simulink model "dVOC_control_demo_fault_2023b_constDC"  (R2023b)
settings: Solver=ode23tb  StartTime=0.0  StopTime=Tend  RelTol=1e-3
values from neighbouring files (symbols this model uses):
  alpha = 1e-1*V_m^2    [dVOC_control_Psensitivity.m]    (also in dVOC_control_demo.m)
  C_4 = 0.1670*C_b    (= 1.00487241952e-06)    [dVOC_control_Psensitivity.m]    (also in dVOC_control_demo.m)
  C_8 = 0.2275*C_b    (= 1.36891302659e-06)    [dVOC_control_Psensitivity.m]    (also in dVOC_control_demo.m)
  C_dc = 0.008*(n)    (= 1.6)    [dVOC_control_Psensitivity.m]    (also in dVOC_control_demo.m)
  C_f = n*300*10^-6    (= 0.06)    [dVOC_control_Psensitivity.m]    (also in dVOC_control_demo.m)
  droop_percentage = 1    [dVOC_control_Psensitivity.m]    (also in dVOC_control_demo.m)
  eta = m_p*V_m^2    [dVOC_control_Psensitivity.m]    (also in dVOC_control_demo.m)
  i_ll = -1.15*(S_b/Vdc_n)-i_loss_dc    [dVOC_control_Psensitivity.m]    (also in dVOC_control_demo.m)
  i_ul = 1.15*(S_b/Vdc_n)+i_loss_dc    [dVOC_control_Psensitivity.m]    (also in dVOC_control_demo.m)
  k_dc = eta_1/(Vdc_n*m_p)    [dVOC_control_Psensitivity.m]    (also in dVOC_control_demo.m)
  K_p = (1/Vdc_n)    [dVOC_control_Psensitivity.m]    (also in dVOC_control_demo.m)
  K_r = 1/R_dc    [dVOC_control_Psensitivity.m]    (also in dVOC_control_demo.m)
  Kff_i = 1    [dVOC_control_Psensitivity.m]    (also in dVOC_control_demo.m)
  Kff_v = 1    [dVOC_control_Psensitivity.m]    (also in dVOC_control_demo.m)
  Ki_i = (1/n)*1.19    (= 0.00595)    [dVOC_control_Psensitivity.m]    (also in dVOC_control_demo.m)
  Ki_v = (n)*1.161022    (= 232.2044)    [dVOC_control_Psensitivity.m]    (also in dVOC_control_demo.m)
  Kp_i = 0.738891    [dVOC_control_Psensitivity.m]    (also in dVOC_control_demo.m)
  Kp_v = 0.52    [dVOC_control_Psensitivity.m]    (also in dVOC_control_demo.m)
  L1_pu = 1*0.0186/m    (= 0.000186)    [dVOC_control_Psensitivity.m]    (also in dVOC_control_demo.m)
  L_45 = L_lines(2)    [dVOC_control_Psensitivity.m]    (also in dVOC_control_demo.m)
  L_89 = L_lines(8)    [dVOC_control_Psensitivity.m]    (also in dVOC_control_demo.m)
  L_94 = L_lines(9)    [dVOC_control_Psensitivity.m]    (also in dVOC_control_demo.m)
  L_f = (1/n)*200*10^-6    (= 1e-06)    [dVOC_control_Psensitivity.m]    (also in dVOC_control_demo.m)
  n = 200    [dVOC_control_Psensitivity.m]    (also in dVOC_control_demo.m)
  pl = S_b*ps    (= 75000000)    [dVOC_control_Psensitivity.m]    (also in dVOC_control_demo.m)
  ps = base/3    (= 0.75)    [dVOC_control_Psensitivity.m]    (also in dVOC_control_demo.m)
  qs = [0;0]    [dVOC_control_Psensitivity.m]    (also in dVOC_control_demo.m)
  R1_pu = 1*0.00734/m    (= 7.34e-05)    [dVOC_control_Psensitivity.m]    (also in dVOC_control_demo.m)
  R_45 = R_lines(2)    [dVOC_control_Psensitivity.m]    (also in dVOC_control_demo.m)
  R_89 = R_lines(8)    [dVOC_control_Psensitivity.m]    (also in dVOC_control_demo.m)
  R_94 = R_lines(9)    [dVOC_control_Psensitivity.m]    (also in dVOC_control_demo.m)
  R_dc = (Vdc_n/(0.05*(S_b)/Vdc_n))    [dVOC_control_Psensitivity.m]    (also in dVOC_control_demo.m)
  R_f = 0.001/n    (= 5e-06)    [dVOC_control_Psensitivity.m]    (also in dVOC_control_demo.m)
  S_b = 100*(10^6)    (= 100000000)    [dVOC_control_Psensitivity.m]    (also in dVOC_control_demo.m)
  S_bt = S_b    (= 100000000)    [dVOC_control_Psensitivity.m]    (also in dVOC_control_demo.m)
  t_disturbance = linspace(0.01,0.2,10)    [dVOC_control_Psensitivity.m]    (also in dVOC_control_demo.m; data_post_process_ExtendSmooth.m = 5+linspace(0.01,0.2,n_period); data_post_process_ExtendSmooth_Psensitivity.m = 5+linspace(0.0,0.0,n_period))
  T_en = T_load(1)-0.5    [dVOC_control_Psensitivity.m]    (also in dVOC_control_demo.m)
  T_load = [5 5]    [dVOC_control_Psensitivity.m]    (also in dVOC_control_demo.m = [5 5.2])
  T_load1 = [T_load(1)-dt_load(1), T_load(1)]    [dVOC_control_Psensitivity.m]    (also in dVOC_control_demo.m = [T_load(1), T_load(1) + dt_load(1)])
  T_load2 = [T_load(1)-dt_load(2), T_load(1)]    [dVOC_control_Psensitivity.m]    (also in dVOC_control_demo.m = [T_load(1), T_load(1) + dt_load(2)])
  T_loss = Tend    (= 8)    [dVOC_control_Psensitivity.m]    (also in dVOC_control_demo.m)
  T_s = 3.125e-4/4    (= 7.8125e-05)    [dVOC_control_Psensitivity.m]    (also in dVOC_control_demo.m)
  tau_dc = 0.05    [dVOC_control_Psensitivity.m]    (also in dVOC_control_demo.m)
  tau_g = 5    [dVOC_control_Psensitivity.m]    (also in dVOC_control_demo.m)
  V1_rms = 1000    [dVOC_control_Psensitivity.m]    (also in dVOC_control_demo.m)
  V2_rms = 13800    [dVOC_control_Psensitivity.m]    (also in dVOC_control_demo.m)
  V_m = sqrt(2/3)*V1_rms    [dVOC_control_Psensitivity.m]    (also in dVOC_control_demo.m)
  Vdc_n = 3*V_m    [dVOC_control_Psensitivity.m]    (also in dVOC_control_demo.m)
  w_b = 2*pi*f_b    (= 314.159265359)    [dVOC_control_Psensitivity.m]    (also in dVOC_control_demo.m)
  w_f = 2*pi*5    (= 31.4159265359)    [dVOC_control_Psensitivity.m]    (also in dVOC_control_demo.m)
undefined symbols (not defined in the file or in its folder): D1, Delta, i_dc, i_t
libraries: eePMU x12, simulink_extras x9, spsabctoAlphaBetaZeroLib x9, spsSeriesRLCBranchLib x8, spsVoltageMeasurementLib x7, spsThreePhaseVIMeasurementLib x6, spsCurrentMeasurementLib x6, spsabctodq0Lib x6, spsGroundLib x5, spsThreePhaseParallelRLCLoadLib x3, spsThreePhaseBreakerLib x3, cstblocks x3
(part 1 of 2)
settings Model: ExtModeTrigDuration=100  Creator=TayyebiA  LastModifiedBy=lab-admin
settings SolverCC: AlgebraicLoopSolver=TrustRegion
settings DataIOCC: SaveFormat=StructureWithTime  SaveOutput=off  ReturnWorkspaceOutputs=off  StateSaveName=tmp_raccel_xout  SignalLoggingName=tmp_raccel_logsout
settings OptimizationCC: EfficientMapNaN2IntZero=off
settings DebuggingCC: AlgebraicLoopMsg=none  ArithmeticOperatorsInVariantConditions=warning
settings HardwareCC: TargetBitPerLong=64  TargetBitPerPointer=64  TargetBitPerSizeT=64  TargetBitPerPtrDiffT=64  TargetLongLongMode=on  TargetIntDivRoundTo=Zero  TargetEndianess=LittleEndian  TargetWordSize=64  TargetHWDeviceType=MATLAB Host  ProdEqTarget=off
settings ModelReferenceCC: EnableRefExpFcnMdlSchedulingChecks=on
settings SFSimCC: SimUseLocalCustomCode=off  CustomCodeUndefinedFunction=UseInterfaceOnly
settings RTWCC: RTWUseLocalCustomCode=off
settings CodeAppCC: MaxIdLength=128
settings GRTTargetCC: TargetLangStandard=C89/C90 (ANSI)  CombineOutputUpdateFcns=off  GRTInterface=on

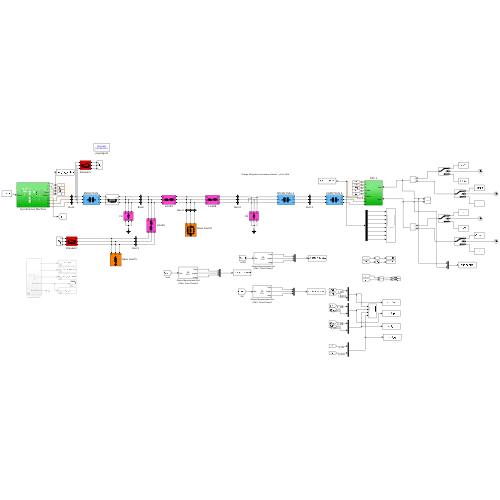
[thumbnail: Simulink's stored preview of the top-level diagram]
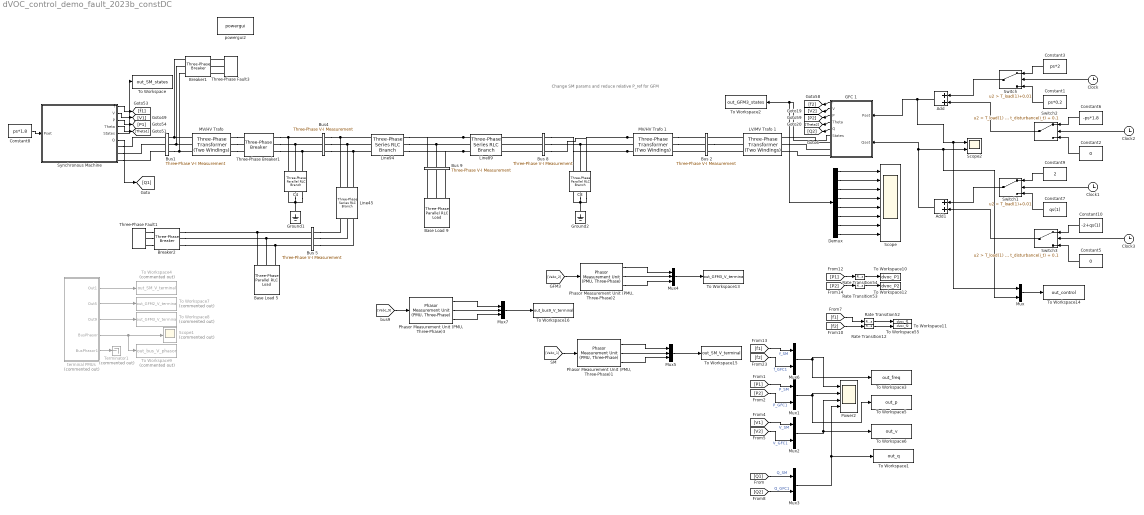
== system dVOC_control_demo_fault_2023b_constDC ==
  note: Change SM params and reduce relative P_ref for GFM
  Add : Sum
  Add1 : Sum
  Base Load 5 : spsThreePhaseParallelRLCLoadLib/Three-Phase Parallel RLC Load  LConnTagsString=A|B|C  Configuration=Y (grounded)  NominalVoltage=230e3  Vabc=[1e3 1e3 1e3]  Vabcp=[1e3 1e3 1e3]  NominalFrequency=50  UnbalancedPower=off  ActivePower=pl  InductivePower=0  CapacitivePower=0  Pabc=[10e3 9e3 11e3]  QLabc=[100 90 110]  QCabc=[100 90 110]  Pabcp=[10e3 9e3 11e3]  QLabcp=[100 90 110]  QCabcp=[100 90 110]  Measurements=None  LoadType=constant Z
  "Base Load 9 " : spsThreePhaseParallelRLCLoadLib/Three-Phase Parallel RLC Load  LConnTagsString=A|B|C  Configuration=Y (grounded)  NominalVoltage=230e3  Vabc=[1e3 1e3 1e3]  Vabcp=[1e3 1e3 1e3]  NominalFrequency=50  UnbalancedPower=off  ActivePower=pl  InductivePower=1*pl  CapacitivePower=1*pl  Pabc=[10e3 9e3 11e3]  QLabc=[100 90 110]  QCabc=[100 90 110]  Pabcp=[10e3 9e3 11e3]  QLabcp=[100 90 110]  QCabcp=[100 90 110]  Measurements=None  LoadType=constant PQ
  Breaker1 : spsThreePhaseBreakerLib/Three-Phase Breaker  InitialState=open  SwitchA=on  SwitchB=on  SwitchC=on  SwitchTimes=[T_load2]  External=off  BreakerResistance=0.01  SnubberResistance=1e6  SnubberCapacitance=inf  Measurements=None
  Breaker2 : spsThreePhaseBreakerLib/Three-Phase Breaker  InitialState=open  SwitchA=on  SwitchB=on  SwitchC=on  SwitchTimes=[T_load1]  External=off  BreakerResistance=0.01  SnubberResistance=1e6  SnubberCapacitance=inf  Measurements=None
  Bus 2 : spsThreePhaseVIMeasurementLib/Three-Phase V-I Measurement  VoltageMeasurement=phase-to-ground  SetLabelV=on  LabelV=Vabc_2  Vpu=on  VpuLL=off  CurrentMeasurement=no  SetLabelI=on  LabelI=Iabc_8  Ipu=on  Pbase=S_b  Vbase=V2_rms  OutputType=Complex  PhasorSimulation=off  PSBequivalent=0
  Bus 5 : spsThreePhaseVIMeasurementLib/Three-Phase V-I Measurement  VoltageMeasurement=phase-to-ground  SetLabelV=on  LabelV=Vabc_5  Vpu=on  VpuLL=off  CurrentMeasurement=no  SetLabelI=on  LabelI=Iabc_5  Ipu=on  Pbase=S_b  Vbase=V_b  OutputType=Complex  PhasorSimulation=off  PSBequivalent=0
  Bus 8 : spsThreePhaseVIMeasurementLib/Three-Phase V-I Measurement  VoltageMeasurement=phase-to-ground  SetLabelV=on  LabelV=Vabc_8  Vpu=on  VpuLL=off  CurrentMeasurement=no  SetLabelI=on  LabelI=Iabc_8  Ipu=on  Pbase=S_b  Vbase=V_b  OutputType=Complex  PhasorSimulation=off  PSBequivalent=0
  Bus 9 : spsThreePhaseVIMeasurementLib/Three-Phase V-I Measurement  VoltageMeasurement=phase-to-ground  SetLabelV=on  LabelV=Vabc_9  Vpu=on  VpuLL=off  CurrentMeasurement=no  SetLabelI=on  LabelI=Iabc_9  Ipu=on  Pbase=S_b  Vbase=V_b  OutputType=Complex  PhasorSimulation=off  PSBequivalent=0
  Bus1 : spsThreePhaseVIMeasurementLib/Three-Phase V-I Measurement  VoltageMeasurement=phase-to-ground  SetLabelV=on  LabelV=Vabc_1  Vpu=on  VpuLL=off  CurrentMeasurement=no  SetLabelI=on  LabelI=Iabc_1  Ipu=on  Pbase=S_b  Vbase=V2_rms  OutputType=Complex  PhasorSimulation=off  PSBequivalent=0
  Bus4 : spsThreePhaseVIMeasurementLib/Three-Phase V-I Measurement  VoltageMeasurement=phase-to-ground  SetLabelV=on  LabelV=Vabc_4  Vpu=on  VpuLL=off  CurrentMeasurement=no  SetLabelI=on  LabelI=Iabc_4  Ipu=on  Pbase=S_b  Vbase=V_b  OutputType=Complex  PhasorSimulation=off  PSBequivalent=0
  C4 : spsThreePhaseParallelRLCBranchLib/Three-Phase Parallel RLC Branch  LConnTagsString=A|B|C  RConnTagsString=A|B|C  BranchType=C  Resistance=1  Inductance=1e-3  Capacitance=C_4  Measurements=None
  C8 : spsThreePhaseParallelRLCBranchLib/Three-Phase Parallel RLC Branch  LConnTagsString=A|B|C  RConnTagsString=A|B|C  BranchType=C  Resistance=1  Inductance=1e-3  Capacitance=C_8  Measurements=None
  Clock{,1..3} (4 alike) : Clock
      settings: Decimation=5
  Constant1 : Constant  Value=ps*0.2
  Constant10 : Constant  Value=-2+qs(1)
  Constant2 : Constant  Value=0
  Constant3 : Constant  Value=ps*2
  Constant5 : Constant  Value=0
  Constant6 : Constant  Value=-ps*1.8
  Constant7 : Constant  Value=qs(1)
  Constant8 : Constant  Value=ps*1.8
  Constant9 : Constant  Value=2
  Demux : Demux  Outputs=8
  GFC 1 : Subsystem
  Ground1 : spsGroundLib/Ground  LConnTagsString=a
  Ground2 : spsGroundLib/Ground  LConnTagsString=a
  LV/MV Trafo 1 : spsThreePhaseTransformerTwoWindingsLib/Three-Phase Transformer (Two Windings)  Winding1Connection=Yg  Winding2Connection=Yg  CoreType=Three single-phase transformers  SetSaturation=off  Hysteresis=off  DataFile='hysteresis'  SetInitialFlux=off  Measurements=None  UNITS=pu  NominalPower=[S_bt 50 ]  Winding1="[ V1_rms R1_pu  L1_pu]"  Winding2=[ V2_rms R1_pu L1_pu]  Rm=Rm_pu  Lm=Lm_pu  L0=0.5  Saturation="[ 0,0  ;  0.005,1.2  ;  1.0,1.4 ]"  InitialFluxes=[ 0.8 , -0.8 , 0.7 ]  BreakLoop=off  DiscreteSolver=Trapezoidal iterative  DataType=off  TransfoNumber=0
  Line45 : spsThreePhaseSeriesRLCBranchLib/Three-Phase Series RLC Branch  LConnTagsString=A|B|C  RConnTagsString=A|B|C  BranchType=RL  Resistance=R_45  Inductance=L_45  Capacitance=0  Measurements=None
  Line89 : spsThreePhaseSeriesRLCBranchLib/Three-Phase Series RLC Branch  LConnTagsString=A|B|C  RConnTagsString=A|B|C  BranchType=RL  Resistance=R_89  Inductance=L_89  Capacitance=0  Measurements=None
  Line94 : spsThreePhaseSeriesRLCBranchLib/Three-Phase Series RLC Branch  LConnTagsString=A|B|C  RConnTagsString=A|B|C  BranchType=RL  Resistance=R_94  Inductance=L_94  Capacitance=0  Measurements=None
  "MV/HV Trafo " : spsThreePhaseTransformerTwoWindingsLib/Three-Phase Transformer (Two Windings)  Winding1Connection=Delta (D1)  Winding2Connection=Yg  CoreType=Three single-phase transformers  SetSaturation=off  Hysteresis=off  DataFile='hysteresis'  SetInitialFlux=off  Measurements=None  UNITS=pu  NominalPower=[ 210e6 50 ]  Winding1="[V2_rms 0.0027  0.08]"  Winding2=[230e3 0.0027 0.08]  Rm=500  Lm=500  L0=0.5  Saturation="[ 0,0  ;  0.005,1.2  ;  1.0,1.4 ]"  InitialFluxes=[ 0.8 , -0.8 , 0.7 ]  BreakLoop=off  DiscreteSolver=Trapezoidal iterative  DataType=off  TransfoNumber=0
  "MV/HV Trafo 1 " : spsThreePhaseTransformerTwoWindingsLib/Three-Phase Transformer (Two Windings)  Winding1Connection=Yg  Winding2Connection=Yg  CoreType=Three single-phase transformers  SetSaturation=off  Hysteresis=off  DataFile='hysteresis'  SetInitialFlux=off  Measurements=None  UNITS=pu  NominalPower=[ 210e6 50 ]  Winding1=[V2_rms 0.0027 0.08]  Winding2=[ 230e3 0.0027 0.08]  Rm=500  Lm=500  L0=0.5  Saturation="[ 0,0  ;  0.005,1.2  ;  1.0,1.4 ]"  InitialFluxes=[ 0.8 , -0.8 , 0.7 ]  BreakLoop=off  DiscreteSolver=Trapezoidal iterative  DataType=off  TransfoNumber=0
  Mux{,1..3,6} (5 alike) : Mux  Inputs=2
  Mux4 : Mux  Inputs=3
  Mux5 : Mux  Inputs=3
  Mux7 : Mux  Inputs=3
  "Phasor Measurement Unit (PMU, Three-Phase)1" : eePMU/Phasor Measurement Unit (PMU, Three-Phase)  frequency=50  Nsr=64  k=1
      settings: LibrarySourceBlock=|
      | ee_sl_lib/Measurements/Phasor Measurement Unit
      | (PMU, Three-Phase)
  "Phasor Measurement Unit (PMU, Three-Phase)2" : eePMU/Phasor Measurement Unit (PMU, Three-Phase)  frequency=50  Nsr=64  k=1
      settings: LibrarySourceBlock=|
      | ee_sl_lib/Measurements/Phasor Measurement Unit
      | (PMU, Three-Phase)
  "Phasor Measurement Unit (PMU, Three-Phase)3" : eePMU/Phasor Measurement Unit (PMU, Three-Phase)  frequency=50  Nsr=64  k=1
      settings: LibrarySourceBlock=|
      | ee_sl_lib/Measurements/Phasor Measurement Unit
      | (PMU, Three-Phase)
  Power2 : Scope  NumInputPorts=4
  Rate Transition{12,52..54} (4 alike) : RateTransition  OutPortSampleTime=T_ms
  Scope : Scope  NumInputPorts=8
  Scope1 : Scope  Commented=on
  Scope2 : Scope  NumInputPorts=2
  Switch : Switch  Criteria=u2 > Threshold  Threshold=T_load(1)+0.01  SaturateOnIntegerOverflow=off  InputSameDT=off
  Switch1 : Switch  Criteria=u2 > Threshold  Threshold=T_load(1)+0.01  SaturateOnIntegerOverflow=off  InputSameDT=off
  Switch2 : Switch  Criteria=u2 > Threshold  Threshold=T_load(1) + t_disturbance(i_t) + 0.1  SaturateOnIntegerOverflow=off  InputSameDT=off
  Switch3 : Switch  Criteria=u2 > Threshold  Threshold=T_load(1) + t_disturbance(i_t) + 0.1  SaturateOnIntegerOverflow=off  InputSameDT=off
  Synchronous Machine : Subsystem
  Terminator1 : Terminator  Commented=on
  Three-Phase Breaker1 : spsThreePhaseBreakerLib/Three-Phase Breaker  InitialState=closed  SwitchA=on  SwitchB=on  SwitchC=on  SwitchTimes=[T_loss]  External=off  BreakerResistance=1  SnubberResistance=1e6  SnubberCapacitance=inf  Measurements=None
  Three-Phase Fault1 : spsThreePhaseFaultLib/Three-Phase Fault  InitialStates=0  FaultA=on  FaultB=on  FaultC=on  GroundFault=on  SwitchTimes=[T_load1]  External=off  SwitchStatus=NaN  FaultResistance=0.001  GroundResistance=0.01  SnubberResistance=1e6  SnubberCapacitance=inf  Measurements=None
  Three-Phase Fault3 : spsThreePhaseFaultLib/Three-Phase Fault  InitialStates=0  FaultA=on  FaultB=on  FaultC=on  GroundFault=on  SwitchTimes=[T_load2]  External=off  SwitchStatus=NaN  FaultResistance=0.001  GroundResistance=0.01  SnubberResistance=1e6  SnubberCapacitance=inf  Measurements=None
  To Workspace : ToWorkspace  VariableName=out_SM_states  SaveFormat=Timeseries  SampleTime=-1
  To Workspace1 : ToWorkspace  VariableName=out_q  SaveFormat=Timeseries  SampleTime=-1
  To Workspace10 : ToWorkspace  VariableName=dvoc_P1  SampleTime=-1
  To Workspace11 : ToWorkspace  VariableName=dvoc_f2  SampleTime=-1
  To Workspace12 : ToWorkspace  VariableName=dvoc_P2  SampleTime=-1
  To Workspace13 : ToWorkspace  VariableName=out_GFM3_V_terminal  SaveFormat=Timeseries  SampleTime=-1
  To Workspace14 : ToWorkspace  VariableName=out_control  SaveFormat=Timeseries  SampleTime=-1
  To Workspace15 : ToWorkspace  VariableName=out_SM_V_terminal  SaveFormat=Timeseries  SampleTime=-1
  To Workspace16 : ToWorkspace  VariableName=out_bus9_V_terminal  SaveFormat=Timeseries  SampleTime=-1
  To Workspace2 : ToWorkspace  VariableName=out_GFM3_states  SaveFormat=Timeseries  SampleTime=-1
  To Workspace3 : ToWorkspace  VariableName=out_freq  SaveFormat=Timeseries  SampleTime=-1
  To Workspace4 : ToWorkspace  Commented=on  VariableName=out_SM_V_terminal  SaveFormat=Timeseries  SampleTime=-1
  To Workspace5 : ToWorkspace  VariableName=out_p  SaveFormat=Timeseries  SampleTime=-1
  To Workspace55 : ToWorkspace  VariableName=dvoc_f1  SampleTime=-1
  To Workspace6 : ToWorkspace  VariableName=out_v  SaveFormat=Timeseries  SampleTime=-1
  To Workspace7 : ToWorkspace  Commented=on  VariableName=out_GFM2_V_terminal  SaveFormat=Timeseries  SampleTime=-1
  To Workspace8 : ToWorkspace  Commented=on  VariableName=out_GFM3_V_terminal  SaveFormat=Timeseries  SampleTime=-1
  To Workspace9 : ToWorkspace  Commented=on  VariableName=out_bus_V_phasor  SaveFormat=Timeseries  SampleTime=-1
  powergui2 : sps_lib/powergui  Priority=1  SimulationMode=Discrete  SampleTime=T_s  frequency=50  Iterations=50  frequencyindice=0  Pbase=100e6  ErrMax=0.0001  UnitsV=kV  UnitsW=MW  buscounter=0  FunctionMessages=off  echomessages=off  EnableUseOfTLC=off  CurrentSourceSwitches=off  DisableSnubberDevices=off  DisableRonSwitches=off  DisableVfSwitches=off  DisplayEquations=off  AutomaticDiscreteSolvers=off  SolverType=Tustin/Backward Euler (TBE)  Interpol=off  ExternalGateDelay=off  methode=off  Ts=100  x0status=blocks  SPID=off  SwTol=0  HookPort=off  NonlinearTolerance=1e-4  nMaxIteration=100  ContinueOnMaxIteration=off  RestoreLinks=warning  ResistiveCurrentMeasurement=off  Frange=[0:2:500]  Ylog=off  Xlog=on  ShowGrid=off  save=off  variable=ZData  structure=0  ZoomFFT=off  StartTime=0.0  cycles=1  DisplayStyle=1  fundamental=60  FreqAxis=off  MaxFrequency=1000  frequencyindicesteady=1  RmsSteady=1  display=off
  terminal PMUs : Subsystem  Commented=on
  wires:
  Constant8/1 -> Synchronous Machine/1(Pset)
  Synchronous Machine/1(f) -> [f1]
  Synchronous Machine/2(V) -> [V1]
  Synchronous Machine/3(P) -> [P1]
  Synchronous Machine/4(Theta) -> [Theta1]
  [f1] -> Mux6/1  "f_SM"
  [f2] -> Mux6/2  "f_GFC1"
  [P1] -> Mux1/1  "P_SM"
  [P2] -> Mux1/2  "P_GFC1"
  [V2] -> Mux2/2  "V_GFC1"
  [V1] -> Mux2/1  "V_SM"
  Mux6/1 -> Power2/1, To Workspace3/1
  Mux1/1 -> Power2/2, To Workspace5/1
  Mux2/1 -> To Workspace6/1, Power2/3
  GFC 1/1(f) -> [f2]
  GFC 1/2(V) -> [V2]
  GFC 1/3(P) -> [P2]
  GFC 1/4(Theta) -> [Theta2]
  GFC 1/5(Q) -> [Q2]
  Mux3/1 -> To Workspace1/1, Power2/4
  [Q2] -> Mux3/2  "Q_GFC1"
  Rate Transition12/1 -> To Workspace11/1
  Rate Transition53/1 -> To Workspace12/1
  Rate Transition54/1 -> To Workspace10/1
  Rate Transition52/1 -> To Workspace55/1
  [f1] -> Rate Transition52/1
  [f2] -> Rate Transition12/1
  [P2] -> Rate Transition53/1
  [P1] -> Rate Transition54/1
  terminal PMUs/3(Out9) -> To Workspace8/1
  terminal PMUs/1(Out1) -> To Workspace4/1
  terminal PMUs/2(Out5) -> To Workspace7/1
  Synchronous Machine/5(States) -> To Workspace/1
  GFC 1/6(States) -> To Workspace2/1, Demux/1
  Demux/1 -> Scope/1
  Demux/2 -> Scope/2
  Demux/3 -> Scope/3
  Demux/4 -> Scope/4
  Demux/5 -> Scope/5
  Demux/6 -> Scope/6
  Demux/7 -> Scope/7
  Demux/8 -> Scope/8
  terminal PMUs/4(BusPhasor) -> To Workspace9/1, Scope1/1
  terminal PMUs/5(BusPhasor1) -> Terminator1/1
  Clock/1 -> Switch/2
  Constant3/1 -> Switch/1
  Constant1/1 -> Switch/3
  Synchronous Machine/6(Q) -> [Q1]
  [Q1] -> Mux3/1  "Q_SM"
  Clock2/1 -> Switch2/2
  Constant2/1 -> Switch2/3
  Constant6/1 -> Switch2/1
  Add/1 -> Mux/1, Scope2/1, GFC 1/1(Pset)
  Switch/1 -> Add/1
  Switch2/1 -> Add/2
  Constant5/1 -> Switch3/3
  Add1/1 -> Mux/2, Scope2/2, GFC 1/2(Qset)
  Switch1/1 -> Add1/1
  Clock3/1 -> Switch3/2
  Switch3/1 -> Add1/2
  Constant10/1 -> Switch3/1
  Constant7/1 -> Switch1/3
  Clock1/1 -> Switch1/2
  Constant9/1 -> Switch1/1
  "Phasor Measurement Unit (PMU, Three-Phase)2"/2 -> Mux4/2
  [Vabc_2] -> "Phasor Measurement Unit (PMU, Three-Phase)2"/1
  "Phasor Measurement Unit (PMU, Three-Phase)2"/1 -> Mux4/1
  "Phasor Measurement Unit (PMU, Three-Phase)2"/3 -> Mux4/3
  Mux4/1 -> To Workspace13/1
  Mux/1 -> To Workspace14/1
  "Phasor Measurement Unit (PMU, Three-Phase)1"/2 -> Mux5/2
  "Phasor Measurement Unit (PMU, Three-Phase)1"/1 -> Mux5/1
  [Vabc_1] -> "Phasor Measurement Unit (PMU, Three-Phase)1"/1
  "Phasor Measurement Unit (PMU, Three-Phase)1"/3 -> Mux5/3
  Mux5/1 -> To Workspace15/1
  "Phasor Measurement Unit (PMU, Three-Phase)3"/2 -> Mux7/2
  [Vabc_9] -> "Phasor Measurement Unit (PMU, Three-Phase)3"/1
  Mux7/1 -> To Workspace16/1
  "Phasor Measurement Unit (PMU, Three-Phase)3"/3 -> Mux7/3
  "Phasor Measurement Unit (PMU, Three-Phase)3"/1 -> Mux7/1
  connections:
  Bus 8/RConn2 -- Line89/RConn2
  "MV/HV Trafo 1 "/RConn3 -- C8/LConn3 -- Bus 8/LConn3
  Line94/RConn2 -- Bus 9/RConn2 -- Line89/LConn2
  Bus 5/LConn3 -- Line45/RConn3
  Line89/LConn1 -- Bus 9/RConn1 -- Line94/RConn1
  C4/RConn2 -- C4/RConn1 -- C4/RConn3 -- Ground1/LConn1
  "MV/HV Trafo 1 "/RConn1 -- C8/LConn1 -- Bus 8/LConn1
  Bus 8/LConn2 -- C8/LConn2 -- "MV/HV Trafo 1 "/RConn2
  C8/RConn3 -- Ground2/LConn1 -- C8/RConn2 -- C8/RConn1
  C4/LConn1 -- Bus4/RConn1 -- Three-Phase Breaker1/RConn1
  Bus4/LConn1 -- Line45/LConn1 -- Line94/LConn1
  Bus4/LConn2 -- Line45/LConn2 -- Line94/LConn2
  Bus 8/RConn3 -- Line89/RConn3
  Bus 8/RConn1 -- Line89/RConn1
  Bus4/RConn3 -- Three-Phase Breaker1/RConn3 -- C4/LConn3
  Bus 5/LConn1 -- Line45/RConn1
  Line89/LConn3 -- Bus 9/RConn3 -- Line94/RConn3
  Bus4/LConn3 -- Line45/LConn3 -- Line94/LConn3
  Bus4/RConn2 -- Three-Phase Breaker1/RConn2 -- C4/LConn2
  Bus 5/LConn2 -- Line45/RConn2
  Base Load 5/LConn3 -- Bus 5/RConn3 -- Breaker2/LConn3
  Base Load 5/LConn1 -- Bus 5/RConn1 -- Breaker2/LConn1
  Base Load 5/LConn2 -- Breaker2/LConn2 -- Bus 5/RConn2
  Bus1/LConn1 -- Breaker1/LConn1 -- "MV/HV Trafo "/LConn1
  Bus1/LConn2 -- Breaker1/LConn2 -- "MV/HV Trafo "/LConn2
  Bus1/LConn3 -- Breaker1/LConn3 -- "MV/HV Trafo "/LConn3
  Synchronous Machine/RConn1 -- Bus1/RConn1
  Synchronous Machine/RConn2 -- Bus1/RConn2
  Synchronous Machine/RConn3 -- Bus1/RConn3
  LV/MV Trafo 1/RConn3 -- Bus 2/LConn3
  "MV/HV Trafo 1 "/LConn2 -- Bus 2/RConn2
  LV/MV Trafo 1/RConn1 -- Bus 2/LConn1
  "MV/HV Trafo 1 "/LConn3 -- Bus 2/RConn3
  "MV/HV Trafo "/RConn1 -- Three-Phase Breaker1/LConn1
  "MV/HV Trafo "/RConn2 -- Three-Phase Breaker1/LConn2
  "MV/HV Trafo "/RConn3 -- Three-Phase Breaker1/LConn3
  GFC 1/RConn3 -- LV/MV Trafo 1/LConn1
  GFC 1/RConn2 -- LV/MV Trafo 1/LConn2
  GFC 1/RConn1 -- LV/MV Trafo 1/LConn3
  Three-Phase Fault1/LConn3 -- Breaker2/RConn3
  Three-Phase Fault1/LConn1 -- Breaker2/RConn1
  Three-Phase Fault1/LConn2 -- Breaker2/RConn2
  Three-Phase Fault3/LConn3 -- Breaker1/RConn3
  Three-Phase Fault3/LConn1 -- Breaker1/RConn1
  Three-Phase Fault3/LConn2 -- Breaker1/RConn2
  Bus 2/RConn1 -- "MV/HV Trafo 1 "/LConn1
  Bus 2/LConn2 -- LV/MV Trafo 1/RConn2
  "Base Load 9 "/LConn3 -- Bus 9/LConn3
  "Base Load 9 "/LConn2 -- Bus 9/LConn2
  "Base Load 9 "/LConn1 -- Bus 9/LConn1

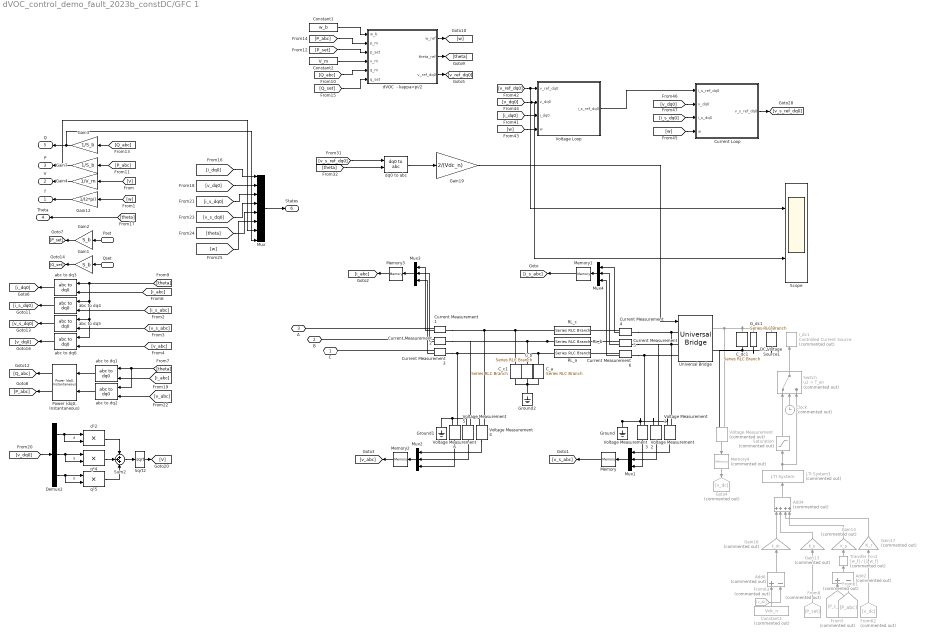
== system dVOC_control_demo_fault_2023b_constDC/GFC 1 ==
  Pset : Inport
  Qset : Inport  Port=2
  Add2 : Sum  Commented=on  Inputs=+-
  Add4 : Sum  Commented=on  Inputs=++++
  Add6 : Sum  Commented=on  Inputs=+-
  C_a : spsSeriesRLCBranchLib/Series RLC Branch  LConnTagsString=__new0  RConnTagsString=__new0  BranchType=C  Resistance=1  Inductance=1e-3  SetiL0=off  InitialCurrent=0  Capacitance=C_f  Setx0=off  InitialVoltage=165  Measurements=None
  C_b : spsSeriesRLCBranchLib/Series RLC Branch  LConnTagsString=__new0  RConnTagsString=__new0  BranchType=C  Resistance=1  Inductance=1e-3  SetiL0=off  InitialCurrent=0  Capacitance=C_f  Setx0=off  InitialVoltage=165  Measurements=None
  C_c1 : spsSeriesRLCBranchLib/Series RLC Branch  LConnTagsString=__new0  RConnTagsString=__new0  BranchType=C  Resistance=1  Inductance=1e-3  SetiL0=off  InitialCurrent=0  Capacitance=C_f  Setx0=off  InitialVoltage=165  Measurements=None
  C_dc1 : spsSeriesRLCBranchLib/Series RLC Branch  LConnTagsString=__new0  RConnTagsString=__new0  BranchType=RC  Resistance=1e-5  Inductance=1e-3  SetiL0=off  InitialCurrent=0  Capacitance=C_dc  Setx0=off  InitialVoltage=Vdc_n  Measurements=None
  Clock : Clock  Commented=on
  Constant1 : Constant  Value=w_b
  Constant2 : Constant  Value=V_m
  Constant3 : Constant  Commented=on  Value=Vdc_n
  Current Loop : Subsystem
  Current Measurement{1..6} (6 alike) : spsCurrentMeasurementLib/Current Measurement  PhasorSimulation=off  OutputType=Complex  PSBequivalent=0
  DC Voltage Source1 : spsDCVoltageSourceLib/DC Voltage Source  Amplitude=Vdc_n  Measurements=None
  Demux2 : Demux  Outputs=3
  From5 : From  Commented=on  GotoTag=P_s_abc
  From61 : From  Commented=on  GotoTag=P_abc
  From62 : From  Commented=on  GotoTag=v_dc
  From63 : From  Commented=on  GotoTag=v_dc
  From8 : From  Commented=on  GotoTag=P_set
  G_dc1 : spsSeriesRLCBranchLib/Series RLC Branch  LConnTagsString=__new0  RConnTagsString=__new0  BranchType=R  Resistance=R_dc  Inductance=1e-3  SetiL0=off  InitialCurrent=0  Capacitance=1e-6  Setx0=off  InitialVoltage=0  Measurements=None
  Gain1 : Gain  Gain=S_b
  Gain12 : Gain  Gain=1/(2*pi)
  Gain13 : Gain  Commented=on  Gain=K_p
  Gain14 : Gain  Commented=on  Gain=K_p
  Gain16 : Gain  Commented=on  Gain=k_dc
  Gain17 : Gain  Commented=on  Gain=K_r
  Gain19 : Gain  Gain=2/(Vdc_n)
  Gain2 : Gain  Gain=S_b
  Gain3 : Gain  Gain=1/S_b
  Gain4 : Gain  Gain=1/V_m
  Gain7 : Gain  Gain=1/S_b
  Goto4 : Goto  Commented=on  GotoTag=v_dc
  Ground : spsGroundLib/Ground  LConnTagsString=a
  Ground1 : spsGroundLib/Ground  LConnTagsString=a
  Ground2 : spsGroundLib/Ground  LConnTagsString=a
  LTI System3 : cstblocks/LTI System  Commented=on  sys=tf(1,[tau_dc 1])  IC=[]  PadeOrder=0
  Memory{,1..3} (4 alike) : Memory
  Memory4 : Memory  Commented=on
  Mux : Mux  Inputs=8
  Mux{1..4} (4 alike) : Mux  Inputs=3
  "Power (dq0, Instantaneous)" : spsPowerdq0InstantaneousLib/Power (dq0, Instantaneous)
      settings: LibrarySourceBlock=|
      | sps_lib/Sensors and Measurements/Power
      | (dq0, Instantaneous)
  RL_a : spsSeriesRLCBranchLib/Series RLC Branch  LConnTagsString=__new0  RConnTagsString=__new0  BranchType=RL  Resistance=R_f  Inductance=L_f  SetiL0=off  InitialCurrent=0  Capacitance=1e-6  Setx0=off  InitialVoltage=0  Measurements=Branch voltage and current
  RL_b : spsSeriesRLCBranchLib/Series RLC Branch  LConnTagsString=__new0  RConnTagsString=__new0  BranchType=RL  Resistance=R_f  Inductance=L_f  SetiL0=off  InitialCurrent=0  Capacitance=1e-6  Setx0=off  InitialVoltage=0  Measurements=None
  RL_c : spsSeriesRLCBranchLib/Series RLC Branch  LConnTagsString=__new0  RConnTagsString=__new0  BranchType=RL  Resistance=R_f  Inductance=L_f  SetiL0=off  InitialCurrent=0  Capacitance=1e-6  Setx0=off  InitialVoltage=0  Measurements=None
  Saturation : Saturate  Commented=on  UpperLimit=i_ul  LowerLimit=i_ll
  Scope : Scope  NumInputPorts=2
  Sqrt2 : Sqrt
  Sum2 : Sum  Inputs=+++  InputSameDT=on  SaturateOnIntegerOverflow=on  OutDataTypeStr=Inherit: Same as first input
  Switch : Switch  Commented=on  Criteria=u2 > Threshold  Threshold=T_en  SaturateOnIntegerOverflow=off  InputSameDT=off
  Transfer Fcn2 : TransferFcn  Commented=on  Numerator=[w_f]  Denominator=[1 w_f]
  Universal Bridge : spsUniversalBridgeLib/Universal Bridge  Arms=3  SnubberResistance=1e5  SnubberCapacitance=inf  Device=Average-model based VSC  Ron=1e-3  Lon=0  ForwardVoltages="[  0  0  ]"  ForwardVoltage=0  GTOparameters=[ 10e-6 , 20e-6 ]  IGBTparameters=[ 1e-6 , 2e-6 ]  Measurements=None  Measurements_2=None  converterType=Rectifier
  Voltage Loop : Subsystem
  Voltage Measurement : spsVoltageMeasurementLib/Voltage Measurement  Commented=on  PhasorSimulation=off  OutputType=Complex  PSBequivalent=0
  Voltage Measurement{1..6} (6 alike) : spsVoltageMeasurementLib/Voltage Measurement  PhasorSimulation=off  OutputType=Complex  PSBequivalent=0
  abc to dq{1..6} (6 alike) : spsabctodq0Lib/abc to dq0  Alignment=90 degrees behind phase A axis
  dVOC  - kappa=pi/2 : Subsystem
  dq0 to abc : spsdq0toabcLib/dq0 to abc  Alignment=90 degrees behind phase A axis
  d²2 : Product  InputSameDT=on  RndMeth=Zero  SaturateOnIntegerOverflow=on  OutDataTypeStr=Inherit: Same as first input
  i_dc1 : spsControlledCurrentSourceLib/Controlled Current Source  Commented=on  Initialize=off  Source_Type=DC  Amplitude=i_dc  Phase=0  Frequency=0  Measurements=None
  q²4 : Product  InputSameDT=on  RndMeth=Zero  SaturateOnIntegerOverflow=on  OutDataTypeStr=Inherit: Same as first input
  q²5 : Product  InputSameDT=on  RndMeth=Zero  SaturateOnIntegerOverflow=on  OutDataTypeStr=Inherit: Same as first input
  C : PMIOPort  Side=Right
  B : PMIOPort  Port=2  Side=Right
  A : PMIOPort  Port=3  Side=Right
  f : Outport  VectorParamsAs1DForOutWhenUnconnected=off
  V : Outport  Port=2  VectorParamsAs1DForOutWhenUnconnected=off
  P : Outport  Port=3  VectorParamsAs1DForOutWhenUnconnected=off
  Theta : Outport  Port=4  VectorParamsAs1DForOutWhenUnconnected=off
  Q : Outport  Port=5  VectorParamsAs1DForOutWhenUnconnected=off
  States : Outport  Port=6  VectorParamsAs1DForOutWhenUnconnected=off
  wires:
  Add4/1 -> LTI System3/1
  Clock/1 -> Switch/2
  Saturation/1 -> Switch/1
  LTI System3/1 -> Switch/3, Saturation/1
  Gain7/1 -> Mux/7, P/1
  [P_abc] -> Gain7/1
  Current Measurement6/1 -> Mux4/3
  Current Measurement5/1 -> Mux4/2
  Current Measurement4/1 -> Mux4/1
  Current Measurement3/1 -> Mux3/3
  Current Measurement2/1 -> Mux3/2
  Current Measurement1/1 -> Mux3/1
  Voltage Measurement4/1 -> Mux2/1
  Voltage Measurement5/1 -> Mux2/2
  Voltage Measurement6/1 -> Mux2/3
  Voltage Measurement3/1 -> Mux1/3
  Voltage Measurement2/1 -> Mux1/2
  Voltage Measurement1/1 -> Mux1/1
  [V] -> Gain4/1
  Gain2/1 -> [P_set]
  Pset/1 -> Gain2/1
  Gain12/1 -> f/1
  [w] -> Gain12/1
  Mux2/1 -> Memory2/1
  Mux3/1 -> Memory3/1
  Mux1/1 -> Memory/1
  abc to dq1/1 -> "Power (dq0, Instantaneous)"/2
  abc to dq2/1 -> "Power (dq0, Instantaneous)"/1
  [theta] -> abc to dq2/2, abc to dq1/2
  [v_abc] -> abc to dq2/1
  "Power (dq0, Instantaneous)"/2 -> [Q_abc]
  "Power (dq0, Instantaneous)"/1 -> [P_abc]
  [i_abc] -> abc to dq1/1
  Gain4/1 -> V/1
  [theta] -> Theta/1
  [i_abc] -> abc to dq3/1
  [i_s_abc] -> abc to dq4/1
  [v_abc] -> abc to dq6/1
  [v_s_abc] -> abc to dq5/1
  [theta] -> abc to dq4/2, abc to dq5/2, abc to dq6/2, abc to dq3/2
  abc to dq3/1 -> [i_dq0]
  abc to dq4/1 -> [i_s_dq0]
  abc to dq5/1 -> [v_s_dq0]
  abc to dq6/1 -> [v_dq0]
  [theta] -> dq0 to abc/2
  q²4/1 -> Sum2/2
  [v_dq0] -> Demux2/1
  q²5/1 -> Sum2/3
  Sum2/1 -> Sqrt2/1
  Demux2/3 -> q²5/1, q²5/2  "0"
  d²2/1 -> Sum2/1
  Demux2/2 -> q²4/1, q²4/2  "q"
  Demux2/1 -> d²2/1, d²2/2  "d"
  Sqrt2/1 -> [V]
  Mux4/1 -> Memory1/1
  Memory2/1 -> [v_abc]
  Memory3/1 -> [i_abc]
  Voltage Measurement/1 -> Memory4/1
  Memory4/1 -> Goto4/1
  Memory/1 -> [v_s_abc]
  Memory1/1 -> [i_s_abc]
  dq0 to abc/1 -> Gain19/1
  [w] -> Current Loop/4(w)
  [v_ref_dq0] -> Scope/1, Voltage Loop/1(v_ref_dq0)
  [i_dq0] -> Voltage Loop/3(i_dq0)
  Voltage Loop/1(i_s_ref_dq0) -> Current Loop/1(i_s_ref_dq0)
  [v_dq0] -> Current Loop/2(v_dq0)
  [i_s_dq0] -> Current Loop/3(i_s_dq0)
  Current Loop/1(v_s_ref_dq0) -> [v_s_ref_dq0]
  [w] -> Voltage Loop/4(w)
  [v_dq0] -> Scope/2, Voltage Loop/2(v_dq0)
  Switch/1 -> i_dc1/1
  Gain19/1 -> Universal Bridge/1
  [v_s_ref_dq0] -> dq0 to abc/1
  Qset/1 -> Gain1/1
  Gain1/1 -> [Q_set]
  [Q_abc] -> Gain3/1
  Gain3/1 -> Mux/8, Q/1
  dVOC  - kappa=pi/2/3(v_ref_dq0) -> [v_ref_dq0]
  Constant2/1 -> dVOC  - kappa=pi/2/4(v_m)
  [P_set] -> dVOC  - kappa=pi/2/3(p_set)
  Constant1/1 -> dVOC  - kappa=pi/2/1(w_b)
  [P_abc] -> dVOC  - kappa=pi/2/2(p_m)
  dVOC  - kappa=pi/2/1(w_ref) -> [w]
  [Q_set] -> dVOC  - kappa=pi/2/6(q_set)
  dVOC  - kappa=pi/2/2(theta_ref) -> [theta]
  [Q_abc] -> dVOC  - kappa=pi/2/5(q_m)
  Add6/1 -> Gain16/1
  From5/1 -> Add2/1
  From61/1 -> Add2/2
  Gain16/1 -> Add4/1
  Constant3/1 -> Add6/1
  From8/1 -> Gain13/1
  Gain17/1 -> Add4/3
  Transfer Fcn2/1 -> Gain14/1
  Gain14/1 -> Add4/4
  From62/1 -> Gain17/1
  Add2/1 -> Transfer Fcn2/1
  From63/1 -> Add6/2
  Gain13/1 -> Add4/2
  [i_dq0] -> Mux/1
  [v_s_dq0] -> Mux/4
  Mux/1 -> States/1
  [i_s_dq0] -> Mux/3
  [theta] -> Mux/5
  [v_dq0] -> Mux/2
  [w] -> Mux/6
  connections:
  RL_b/RConn1 -- Voltage Measurement5/LConn1 -- Current Measurement2/LConn1 -- C_b/LConn1
  Voltage Measurement6/LConn1 -- Current Measurement3/LConn1 -- C_a/LConn1 -- RL_a/RConn1
  Current Measurement4/RConn1 -- RL_c/LConn1
  Current Measurement6/RConn1 -- RL_a/LConn1
  Current Measurement5/RConn1 -- RL_b/LConn1
  Voltage Measurement/LConn1 -- DC Voltage Source1/RConn1 -- G_dc1/LConn1 -- C_dc1/LConn1 -- Universal Bridge/RConn1
  Voltage Measurement6/LConn2 -- Voltage Measurement5/LConn2 -- Voltage Measurement4/LConn2 -- Ground1/LConn1
  Ground/LConn1 -- Voltage Measurement2/LConn2 -- Voltage Measurement1/LConn2 -- Voltage Measurement3/LConn2
  Current Measurement3/RConn1 -- C/RConn1
  Current Measurement2/RConn1 -- B/RConn1
  Current Measurement1/RConn1 -- A/RConn1
  Current Measurement6/LConn1 -- Universal Bridge/LConn3 -- Voltage Measurement3/LConn1
  Universal Bridge/LConn2 -- Current Measurement5/LConn1 -- Voltage Measurement2/LConn1
  Universal Bridge/LConn1 -- Current Measurement4/LConn1 -- Voltage Measurement1/LConn1
  Universal Bridge/RConn2 -- Voltage Measurement/LConn2 -- DC Voltage Source1/LConn1 -- G_dc1/RConn1 -- C_dc1/RConn1
  C_b/RConn1 -- C_a/RConn1 -- Ground2/LConn1 -- C_c1/RConn1
  Voltage Measurement4/LConn1 -- Current Measurement1/LConn1 -- C_c1/LConn1 -- RL_c/RConn1

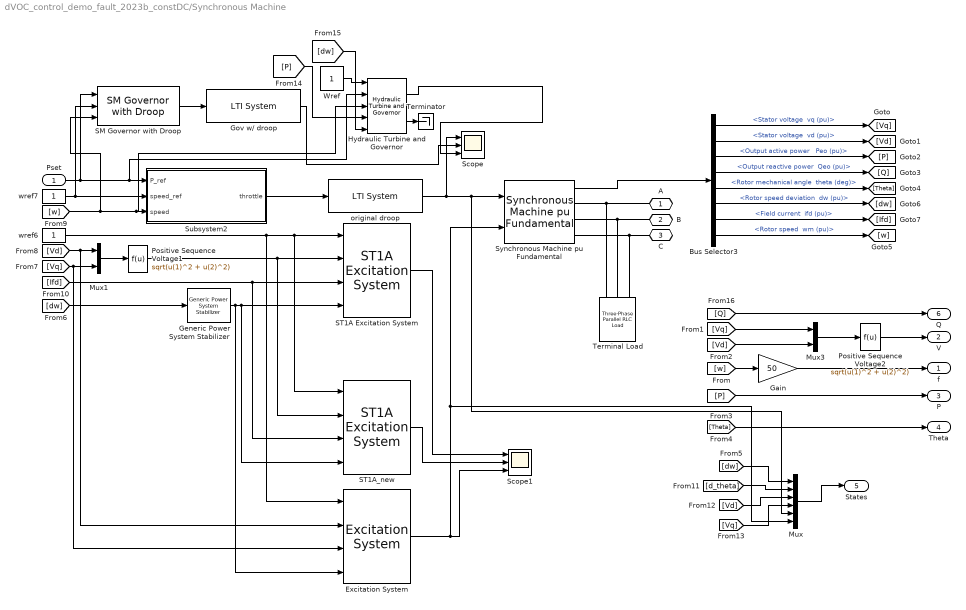
== system dVOC_control_demo_fault_2023b_constDC/Synchronous Machine ==
  Pset : Inport
  Bus Selector3 : BusSelector  OutputSignals="dq0 components.Stator voltage  vq (pu),dq0 components.Stator voltage  vd (pu),Output active power   Peo (pu),Output reactive power  Qeo (pu),Mechanical.Rotor mechanical angle  theta (deg),Mechanical.Rotor speed deviation  dw (pu),dq0 components.Field current  ifd (pu),Mechanical.Rotor speed  wm (pu)"
  Excitation System : spsExcitationSystemLib/Excitation System  tr=20e-3  reg=[ 300, 0.001 ]  exc=[ 1, 0 ]  tgr=[ 0, 0 ]  damp=[ 0.001, 0.1 ]  sat=[ 0, 0 ]  lim=[ -11.5, 11.5, 0 ]  v0="[1.0  1.28]"
      settings: LibrarySourceBlock=sps_lib/Electrical Machines/Synchronous Machine Control/Excitation System
  Gain : Gain  Gain=50
  Generic Power System Stabilizer : spsGenericPowerSystemStabilizerLib/Generic Power System Stabilizer  Tsensor=30e-4  K=2.5  Twashout=2  Tleadlag1=[2*50e-3 0.1*20e-3]  Tleadlag2=[2*3 0.1*5.4]  VSlimits=2*[-0.15 0.15]  Vinit=0  Plot_On=off  MagdB_On=on  FreqRange=logspace(-2,2,500)
      settings: LibrarySourceBlock=|
      | sps_lib/Electrical Machines/Synchronous Machine Control/Generic
      | Power System Stabilizer
  Gov w/ droop : cstblocks/LTI System  sys=ss(-1/tau_g,1/tau_g,1,[])  IC=ps  PadeOrder=0
  Hydraulic Turbine and Governor : spsHydraulicTurbineandGovernorLib/Hydraulic Turbine and Governor  sm="[ 10/3  0.07 ]"  gate="[  0.01  0.97518  -0.1  0.1 ]"  reg="[  0.05*0.1  1.163*4  0.105*4  0  0.01  ]"  hyd="[  0  2.67  ]"  dref=0  po=0.7516
      settings: LibrarySourceBlock=|
      | sps_lib/Electrical Machines/Synchronous Machine Control/Hydraulic Turbine
      | and Governor
  Mux : Mux  Inputs=6
  Mux1 : Mux  Inputs=2
  Mux3 : Mux  Inputs=2
  Positive Sequence Voltage1 : Fcn  Expr=sqrt(u(1)^2 + u(2)^2)
  Positive Sequence Voltage2 : Fcn  Expr=sqrt(u(1)^2 + u(2)^2)
  SM Governor with Droop : eeSmGovernor/SM Governor with Droop  droop_percentage=5  T_G=0.2  pu_throttle0=0.5
      settings: LibrarySourceBlock=|
      | ee_sl_lib/SM Control/SM Governor
      | with Droop
  ST1A Excitation System : spsST1AExcitationSystemLib/ST1A Excitation System  Tr=20e-3  KaTa=[210 0.001]  VIminmax=[-999 +999]  VAminmax=[-999 999]  VRminmax=[-6.0 6.43]  KfTf=[0.001 1]  TbTc=[0 0 0 0]  KLR=1  ILR=2  Kc=0.038  v0=[1 1]  TsBlock=0
      settings: LibrarySourceBlock=|
      | sps_lib/Electrical Machines/Synchronous Machine Control/ST1A
      | Excitation System
  ST1A_new : spsST1AExcitationSystemLib/ST1A Excitation System  Tr=20e-3  KaTa=[210 0.001]  VIminmax=[-999 +999]  VAminmax=[-999 999]  VRminmax=[-6.0 6.43]  KfTf=[0.001*10 1]  TbTc=[0 0 0 0]  KLR=1  ILR=2  Kc=0.038  v0=[1 1]  TsBlock=0
      settings: LibrarySourceBlock=|
      | sps_lib/Electrical Machines/Synchronous Machine Control/ST1A
      | Excitation System
  Scope : Scope  NumInputPorts=3
  Scope1 : Scope  NumInputPorts=3
  Subsystem2 : Subsystem
  Synchronous Machine pu Fundamental : spsSynchronousMachinepuFundamentalLib/Synchronous Machine pu Fundamental  PresetModel=No  MechanicalLoad=Mechanical power Pm  ShowDetailedParameters=on  RotorType=Salient-pole  Units=per unit fundamental parameters  MeasurementBus=off  NominalParameters="[100E6  V2_rms   50]"  Stator="[ 2.85E-03  0.114  1.19  0.36 ]"  Field="[ 5.79E-04  0.114]"  Dampers2=[0.0652, 0.5134, 0.0287, 0.2553, 7.765e-3, 0.9167 ]  Dampers1="[ 1.17E-02  0.182  1.97E-02  0.384 ]"  Mechanical=[ 3.7*.5 0 20]  PolePairs=20  InitialConditions="[ 0  0  0  0  0  0  0  0  1 ]"  SetSaturation=off  Saturation=[0.6404,0.7127,0.8441,0.9214,0.9956,1.082,1.19,1.316,1.457;0.7,0.7698,0.8872,0.9466,0.9969,1.046,1.1,1.151,1.201]  LoadFlowParameters=[1,0,0,0,0]  TsPowergui=0  TsBlock=-1  IterativeModel=Trapezoidal non iterative  IterativeDiscreteModel=Trapezoidal non iterative  BusType=PV  Pref=0  Qref=0  Qmin=-inf  Qmax=inf  PLF=0  QLF=0
      settings: LibrarySourceBlock=|
      | sps_lib/Electrical Machines/Synchronous Machine
      | pu Fundamental
  Terminal Load : spsThreePhaseParallelRLCLoadLib/Three-Phase Parallel RLC Load  LConnTagsString=A|B|C  Configuration=Y (grounded)  NominalVoltage=V2_rms  Vabc=[1e3 1e3 1e3]  Vabcp=[1e3 1e3 1e3]  NominalFrequency=50  UnbalancedPower=off  ActivePower=1  InductivePower=0  CapacitivePower=0  Pabc=[10e3 9e3 11e3]  QLabc=[100 90 110]  QCabc=[100 90 110]  Pabcp=[10e3 9e3 11e3]  QLabcp=[100 90 110]  QCabcp=[100 90 110]  Measurements=None  LoadType=constant Z
  Terminator : Terminator
  Wref : Constant
  original droop : cstblocks/LTI System  sys=ss(-1/tau_g,1/tau_g,1,[])  IC=ps  PadeOrder=0
  wref6 : Constant
  wref7 : Constant
  A : PMIOPort  Side=Right
  B : PMIOPort  Port=2  Side=Right
  C : PMIOPort  Port=3  Side=Right
  f : Outport  VectorParamsAs1DForOutWhenUnconnected=off
  V : Outport  Port=2  VectorParamsAs1DForOutWhenUnconnected=off
  P : Outport  Port=3  VectorParamsAs1DForOutWhenUnconnected=off
  Theta : Outport  Port=4  VectorParamsAs1DForOutWhenUnconnected=off
  States : Outport  Port=5
  Q : Outport  Port=6
  wires:
  Gain/1 -> f/1
  Pset/1 -> SM Governor with Droop/1, Hydraulic Turbine and Governor/2, Subsystem2/1(P_ref)
  Positive Sequence Voltage2/1 -> V/1
  wref7/1 -> Subsystem2/2(speed_ref), SM Governor with Droop/2
  wref6/1 -> Excitation System/1, ST1A_new/1, ST1A Excitation System/1
  Mux3/1 -> Positive Sequence Voltage2/1
  Synchronous Machine pu Fundamental/1 -> Bus Selector3/1
  [w] -> Gain/1
  [Vq] -> Mux3/1
  [Vd] -> Mux3/2
  [P] -> P/1
  [Theta] -> Theta/1
  [w] -> SM Governor with Droop/3, Hydraulic Turbine and Governor/3, Subsystem2/3(speed)
  Subsystem2/1(throttle) -> original droop/1
  Bus Selector3/1 -> [Vq]  "<Stator voltage  vq (pu)>"
  Bus Selector3/2 -> [Vd]  "<Stator voltage  vd (pu)>"
  Bus Selector3/3 -> [P]  "<Output active power   Peo (pu)>"
  Bus Selector3/4 -> [Q]  "<Output reactive power  Qeo (pu)>"
  Bus Selector3/5 -> [Theta]  "<Rotor mechanical angle  theta (deg)>"
  Bus Selector3/6 -> [dw]  "<Rotor speed deviation  dw (pu)>"
  Bus Selector3/7 -> [Ifd]  "<Field current  ifd (pu)>"
  Bus Selector3/8 -> [w]  "<Rotor speed  wm (pu)>"
  original droop/1 -> Mux/5, Synchronous Machine pu Fundamental/1, Scope/1
  Generic Power System Stabilizer/1 -> Excitation System/4, ST1A_new/4, ST1A Excitation System/4
  [dw] -> Generic Power System Stabilizer/1
  [Ifd] -> ST1A Excitation System/3, ST1A_new/3
  Mux1/1 -> Positive Sequence Voltage1/1
  [Vd] -> Excitation System/2, Mux1/1
  [Vq] -> Excitation System/3, Mux1/2
  Positive Sequence Voltage1/1 -> ST1A_new/2, ST1A Excitation System/2
  ST1A Excitation System/1 -> Scope1/1
  [Vd] -> Mux/3
  [Vq] -> Mux/4
  [dw] -> Mux/1
  Mux/1 -> States/1
  [d_theta] -> Mux/2
  SM Governor with Droop/1 -> Gov w/ droop/1
  Gov w/ droop/1 -> Scope/2
  Wref/1 -> Hydraulic Turbine and Governor/1
  [P] -> Hydraulic Turbine and Governor/4
  [dw] -> Hydraulic Turbine and Governor/5
  Hydraulic Turbine and Governor/2 -> Terminator/1
  Hydraulic Turbine and Governor/1 -> Scope/3
  ST1A_new/1 -> Scope1/2
  Excitation System/1 -> Mux/6, Synchronous Machine pu Fundamental/2, Scope1/3
  [Q] -> Q/1
  connections:
  Terminal Load/LConn1 -- Synchronous Machine pu Fundamental/RConn1 -- A/RConn1
  Terminal Load/LConn3 -- Synchronous Machine pu Fundamental/RConn3 -- C/RConn1
  Terminal Load/LConn2 -- Synchronous Machine pu Fundamental/RConn2 -- B/RConn1

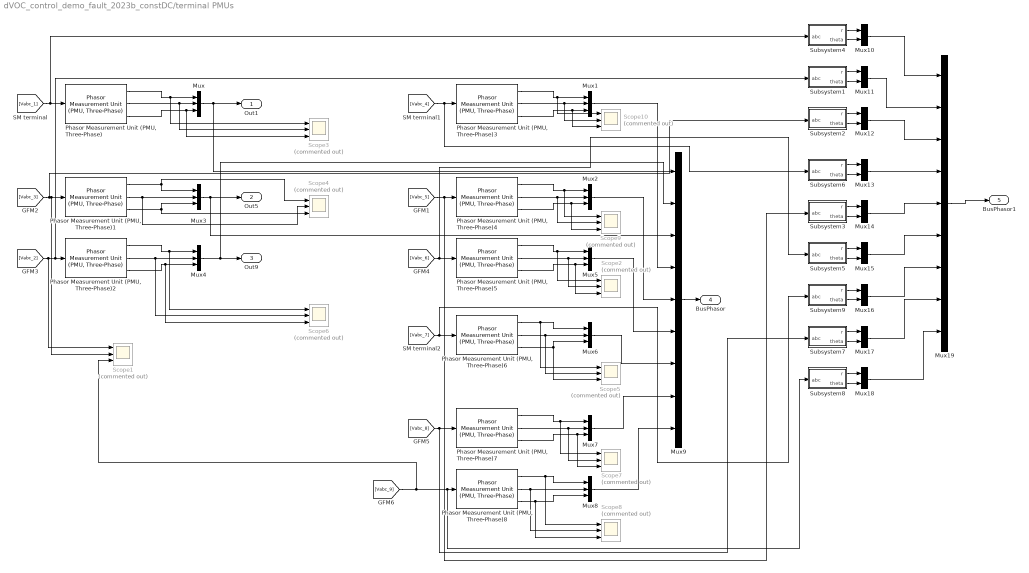
== system dVOC_control_demo_fault_2023b_constDC/terminal PMUs ==
  Mux{,1..8} (9 alike) : Mux  Inputs=3
  Mux{10..18} (9 alike) : Mux  Inputs=2
  Mux19 : Mux  Inputs=9
  Mux9 : Mux  Inputs=9
  Phasor Measurement Unit (PMU, Three-Phase){,1..8} (9 alike) : eePMU/Phasor Measurement Unit (PMU, Three-Phase)  frequency=50  Nsr=64  k=1
      settings: LibrarySourceBlock=|
      | ee_sl_lib/Measurements/Phasor Measurement Unit
      | (PMU, Three-Phase)
  Scope{1..10} (10 alike) : Scope  Commented=on  NumInputPorts=3
  Subsystem1 : Subsystem
  Subsystem2 : Subsystem
  Subsystem3 : Subsystem
  Subsystem4 : Subsystem
  Subsystem5 : Subsystem
  Subsystem6 : Subsystem
  Subsystem7 : Subsystem
  Subsystem8 : Subsystem
  Subsystem9 : Subsystem
  Out1 : Outport
  Out5 : Outport  Port=2
  Out9 : Outport  Port=3
  BusPhasor : Outport  Port=4
  BusPhasor1 : Outport  Port=5
  wires:
  [Vabc_1] -> Subsystem4/1(abc), "Phasor Measurement Unit (PMU, Three-Phase)"/1
  Mux3/1 -> Mux9/3, Out5/1
  "Phasor Measurement Unit (PMU, Three-Phase)1"/3 -> Scope4/3, Mux3/3
  "Phasor Measurement Unit (PMU, Three-Phase)2"/2 -> Scope6/2, Mux4/2
  Mux4/1 -> Mux9/2, Out9/1
  Mux/1 -> Mux9/1, Out1/1
  "Phasor Measurement Unit (PMU, Three-Phase)2"/3 -> Scope6/3, Mux4/3
  "Phasor Measurement Unit (PMU, Three-Phase)"/1 -> Scope3/1, Mux/1
  "Phasor Measurement Unit (PMU, Three-Phase)"/3 -> Scope3/3, Mux/3
  "Phasor Measurement Unit (PMU, Three-Phase)1"/2 -> Scope4/2, Mux3/2
  [Vabc_2] -> Scope1/1, Subsystem1/1(abc), "Phasor Measurement Unit (PMU, Three-Phase)2"/1
  "Phasor Measurement Unit (PMU, Three-Phase)"/2 -> Scope3/2, Mux/2
  "Phasor Measurement Unit (PMU, Three-Phase)2"/1 -> Scope6/1, Mux4/1
  "Phasor Measurement Unit (PMU, Three-Phase)1"/1 -> Scope4/1, Mux3/1
  "Phasor Measurement Unit (PMU, Three-Phase)4"/1 -> Scope9/1, Mux2/1
  "Phasor Measurement Unit (PMU, Three-Phase)3"/3 -> Scope10/3, Mux1/3
  "Phasor Measurement Unit (PMU, Three-Phase)4"/3 -> Scope9/3, Mux2/3
  "Phasor Measurement Unit (PMU, Three-Phase)3"/2 -> Scope10/2, Mux1/2
  [Vabc_6] -> Subsystem5/1(abc), "Phasor Measurement Unit (PMU, Three-Phase)5"/1
  Mux5/1 -> Mux9/6
  Mux1/1 -> Mux9/4
  [Vabc_4] -> Subsystem6/1(abc), "Phasor Measurement Unit (PMU, Three-Phase)3"/1
  "Phasor Measurement Unit (PMU, Three-Phase)3"/1 -> Scope10/1, Mux1/1
  Mux2/1 -> Mux9/5
  "Phasor Measurement Unit (PMU, Three-Phase)4"/2 -> Scope9/2, Mux2/2
  [Vabc_5] -> Subsystem3/1(abc), "Phasor Measurement Unit (PMU, Three-Phase)4"/1
  "Phasor Measurement Unit (PMU, Three-Phase)5"/3 -> Scope2/3, Mux5/3
  "Phasor Measurement Unit (PMU, Three-Phase)5"/1 -> Scope2/1, Mux5/1
  [Vabc_7] -> Subsystem9/1(abc), "Phasor Measurement Unit (PMU, Three-Phase)6"/1
  Mux8/1 -> Mux9/9
  "Phasor Measurement Unit (PMU, Three-Phase)8"/3 -> Scope8/3, Mux8/3
  Mux7/1 -> Mux9/8
  "Phasor Measurement Unit (PMU, Three-Phase)7"/2 -> Scope7/2, Mux7/2
  "Phasor Measurement Unit (PMU, Three-Phase)8"/1 -> Scope8/1, Mux8/1
  "Phasor Measurement Unit (PMU, Three-Phase)6"/2 -> Scope5/2, Mux6/2
  Mux6/1 -> Mux9/7
  "Phasor Measurement Unit (PMU, Three-Phase)8"/2 -> Scope8/2, Mux8/2
  [Vabc_8] -> Subsystem7/1(abc), "Phasor Measurement Unit (PMU, Three-Phase)7"/1
  "Phasor Measurement Unit (PMU, Three-Phase)7"/3 -> Scope7/3, Mux7/3
  "Phasor Measurement Unit (PMU, Three-Phase)6"/3 -> Scope5/3, Mux6/3
  "Phasor Measurement Unit (PMU, Three-Phase)7"/1 -> Scope7/1, Mux7/1
  "Phasor Measurement Unit (PMU, Three-Phase)6"/1 -> Scope5/1, Mux6/1
  Mux9/1 -> BusPhasor/1
  [Vabc_3] -> Scope1/2, "Phasor Measurement Unit (PMU, Three-Phase)1"/1, Subsystem2/1(abc)
  Subsystem4/2(theta) -> Mux10/2
  Subsystem4/1(r) -> Mux10/1
  Subsystem1/2(theta) -> Mux11/2
  Subsystem1/1(r) -> Mux11/1
  Subsystem2/2(theta) -> Mux12/2
  Subsystem2/1(r) -> Mux12/1
  Subsystem3/2(theta) -> Mux14/2
  Subsystem6/2(theta) -> Mux13/2
  Subsystem5/2(theta) -> Mux15/2
  Subsystem3/1(r) -> Mux14/1
  Subsystem6/1(r) -> Mux13/1
  Subsystem5/1(r) -> Mux15/1
  Subsystem7/2(theta) -> Mux17/2
  Subsystem9/2(theta) -> Mux16/2
  Subsystem8/2(theta) -> Mux18/2
  Subsystem7/1(r) -> Mux17/1
  Subsystem9/1(r) -> Mux16/1
  Subsystem8/1(r) -> Mux18/1
  Mux10/1 -> Mux19/1
  Mux11/1 -> Mux19/2
  Mux12/1 -> Mux19/3
  Mux13/1 -> Mux19/4
  Mux14/1 -> Mux19/5
  Mux15/1 -> Mux19/6
  Mux16/1 -> Mux19/7
  Mux17/1 -> Mux19/8
  Mux18/1 -> Mux19/9
  Mux19/1 -> BusPhasor1/1
  [Vabc_9] -> Scope1/3, Subsystem8/1(abc), "Phasor Measurement Unit (PMU, Three-Phase)8"/1
  "Phasor Measurement Unit (PMU, Three-Phase)5"/2 -> Scope2/2, Mux5/2

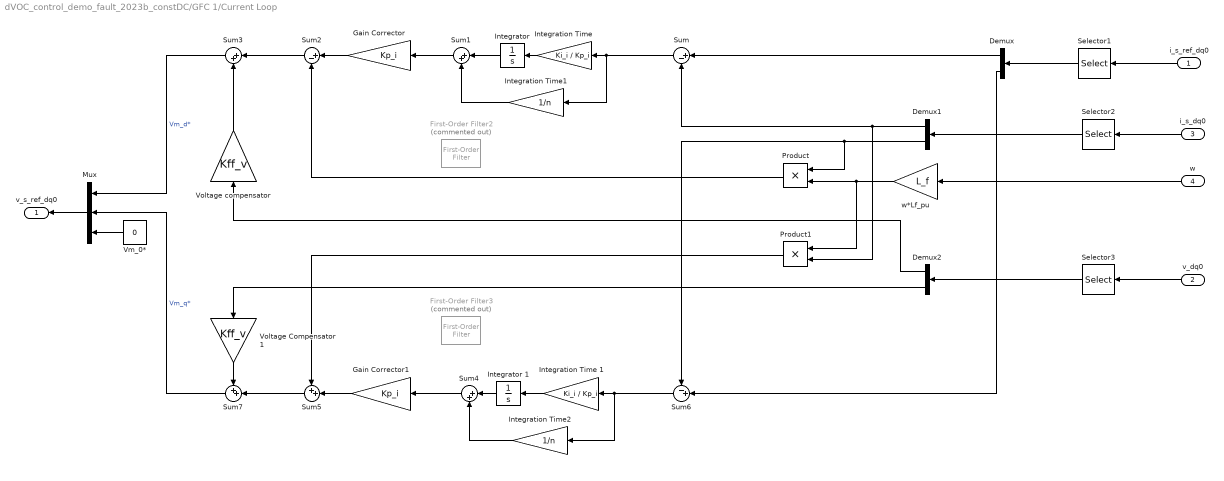
== system dVOC_control_demo_fault_2023b_constDC/GFC 1/Current Loop ==
  i_s_ref_dq0 : Inport
  v_dq0 : Inport  Port=2
  i_s_dq0 : Inport  Port=3
  w : Inport  Port=4
  Demux : Demux  Outputs=2
  Demux1 : Demux  Outputs=2
  Demux2 : Demux  Outputs=2
  First-Order Filter2 : spsFirstOrderFilterLib/First-Order Filter  Commented=on  FilterType=Lowpass  Tc=25e-3  Ts=0  Initialize=on  Vac_Init=[0, 0, 50]  Vdc_Init=1  PlotResponse=off  FreqRange="[0,  200,  1]"
  First-Order Filter3 : spsFirstOrderFilterLib/First-Order Filter  Commented=on  FilterType=Lowpass  Tc=25e-3  Ts=0  Initialize=on  Vac_Init=[0, 0, 50]  Vdc_Init=0  PlotResponse=off  FreqRange="[0,  200,  1]"
  Gain Corrector : Gain  Gain=Kp_i
  Gain Corrector1 : Gain  Gain=Kp_i
  Integration Time : Gain  Gain=Ki_i / Kp_i
  Integration Time 1 : Gain  Gain=Ki_i / Kp_i
  Integration Time1 : Gain  Gain=1/n
  Integration Time2 : Gain  Gain=1/n
  Integrator : Integrator
  Integrator 1 : Integrator
  Mux : Mux  Inputs=3
  Product : Product  RndMeth=Zero
  Product1 : Product  RndMeth=Zero
  Selector1 : Selector  InputPortWidth=3  IndexOptions=Index vector (dialog)  Indices=[1 2]  OutputSizes=1
  Selector2 : Selector  InputPortWidth=3  IndexOptions=Index vector (dialog)  Indices=[1 2]  OutputSizes=1
  Selector3 : Selector  InputPortWidth=3  IndexOptions=Index vector (dialog)  Indices=[1 2]  OutputSizes=1
  Sum : Sum  Inputs=|+-
  Sum1 : Sum  Inputs=|++
  Sum2 : Sum  Inputs=|+-
  Sum3 : Sum  Inputs=|++
  Sum4 : Sum  Inputs=|++
  Sum5 : Sum  Inputs=++|
  Sum6 : Sum  Inputs=-+|
  Sum7 : Sum  Inputs=++|
  Vm_0* : Constant  Value=0
  Voltage Compensator 1 : Gain  Gain=Kff_v
  Voltage compensator : Gain  Gain=Kff_v
  w*Lf_pu : Gain  Gain=L_f
  v_s_ref_dq0 : Outport  VectorParamsAs1DForOutWhenUnconnected=off
  wires:
  Sum/1 -> Integration Time/1, Integration Time1/1
  Integration Time 1/1 -> Integrator 1/1
  Integration Time/1 -> Integrator/1
  Sum5/1 -> Sum7/2
  Sum6/1 -> Integration Time 1/1, Integration Time2/1
  Demux/1 -> Sum/1
  Sum3/1 -> Mux/1  "Vm_d*"
  Sum7/1 -> Mux/2  "Vm_q*"
  Demux2/2 -> Voltage Compensator 1/1
  Voltage Compensator 1/1 -> Sum7/1
  Product/1 -> Sum2/2
  w*Lf_pu/1 -> Product1/1, Product/2
  i_s_ref_dq0/1 -> Selector1/1
  v_dq0/1 -> Selector3/1
  Integrator 1/1 -> Sum4/1
  Voltage compensator/1 -> Sum3/2
  Sum1/1 -> Gain Corrector/1
  Sum2/1 -> Sum3/1
  Sum4/1 -> Gain Corrector1/1
  Demux/2 -> Sum6/2
  Selector1/1 -> Demux/1
  Gain Corrector/1 -> Sum2/1
  w/1 -> w*Lf_pu/1
  Mux/1 -> v_s_ref_dq0/1
  Selector2/1 -> Demux1/1
  i_s_dq0/1 -> Selector2/1
  Selector3/1 -> Demux2/1
  Demux1/2 -> Product/1, Sum6/1
  Vm_0*/1 -> Mux/3
  Integrator/1 -> Sum1/1
  Demux1/1 -> Product1/2, Sum/2
  Demux2/1 -> Voltage compensator/1
  Product1/1 -> Sum5/1
  Gain Corrector1/1 -> Sum5/2
  Integration Time1/1 -> Sum1/2
  Integration Time2/1 -> Sum4/2
